simulink model "SimulinkModel"  (R2021b)
settings: Solver=VariableStepAuto  StartTime=0.0  StopTime=20  RelTol=1e-3
values from neighbouring files (symbols this model uses):
  A = [[0 1 0] ... (first row only)    [Hinfmodel.m]    (also in LQGModel.m = [[0 1]; Model.m = [[0 1]; NewModel.m)
  B = [[0] ... (first row only)    [Hinfmodel.m]    (also in LQGModel.m = [-0.07528015464; Model.m = [0; NewModel.m)
  C = [[1/40.33*0.9 0 0] ... (first row only)    [Hinfmodel.m]    (also in LQGModel.m = [[0.6 0]; Model.m = [[1 0]; NewModel.m)
  D = [0;0;0]    [Hinfmodel.m]    (also in LQGModel.m = [0; Model.m = [0; NewModel.m)
  K = [-0.3972  -0.8279]    [DampingExperiments.m]    (also in LQGModel.m = place(A,B,[-0.2 + 0.1i -0.2-0.1i]); Model.m = place(A,B,[-0.2 + 0.1i -0.2-0.1i]))
settings Model: Creator=willi  LastModifiedBy=willi

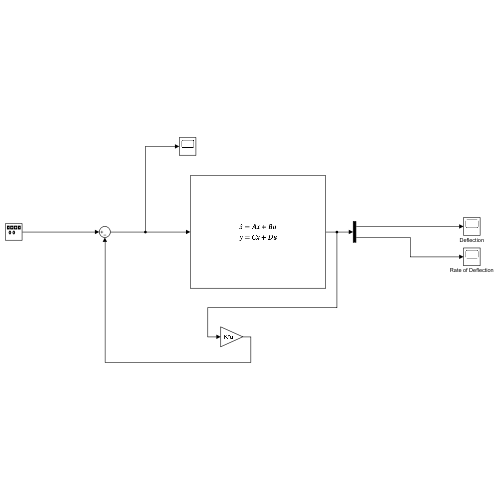
[thumbnail: Simulink's stored preview of the top-level diagram]
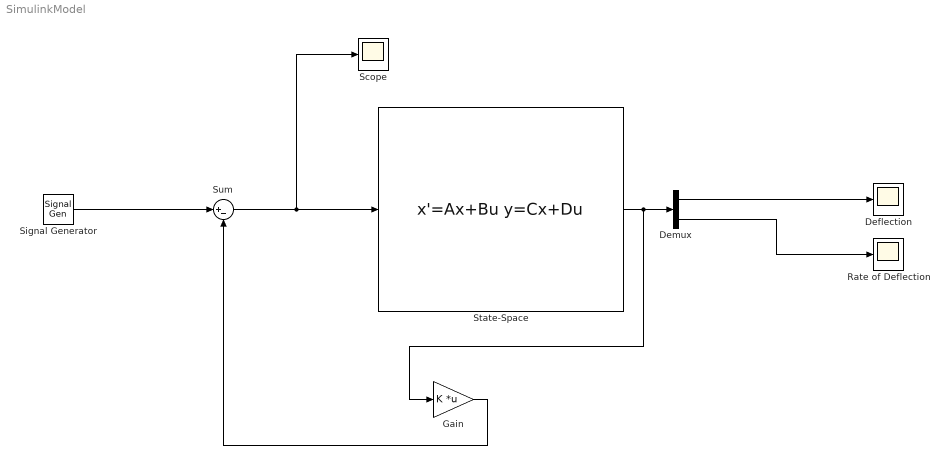
== system SimulinkModel ==
  Deflection : Scope
  Demux : Demux  Outputs=2
  Gain : Gain  Gain=K  Multiplication=Matrix(K*u)
  Rate of Deflection : Scope
  Scope : Scope
  Signal Generator : SignalGenerator  Frequency=20  Units=rad/sec
  State-Space : StateSpace  A=A  B=B  C=C  D=D  InitialCondition=0  ParameterTunability=Unconstrained  ContinuousStateAttributes='sys.StateName'
  Sum : Sum  Inputs=|+-
  wires:
  Signal Generator/1 -> Sum/1
  State-Space/1 -> Gain/1, Demux/1
  Demux/1 -> Deflection/1
  Demux/2 -> Rate of Deflection/1
  Sum/1 -> Scope/1, State-Space/1
  Gain/1 -> Sum/2
